simulink model "mpsk"  (Simulink 6.4)
settings: Solver=FixedStepDiscrete  StartTime=0.0  StopTime=inf  RelTol=1e-3
libraries: commsink2 x2, commdigbbndpm3 x2, commchan3 x1, commrandsrc2 x1
settings Model: Creator=ALEX  LastModifiedBy=student
settings OptimizationCC: InitFltsAndDblsToZero=off
settings DebuggingCC: SignalResolutionControl=UseLocalSettings  MultiTaskDSMMsg=error  MultiTaskCondExecSysMsg=error
settings GRTTargetCC: TargetFcnLib=ansi_tfl_table_tmw.mat

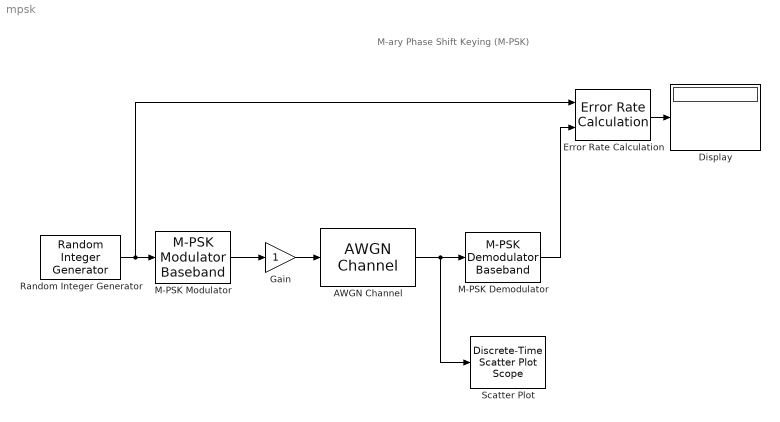
== system mpsk ==
  note: M-ary Phase Shift Keying (M-PSK)
  AWGN Channel : commchan3/AWGN Channel  SystemSampleTime=-1  seed=67  noiseMode="Signal to noise ratio  (Es/No)"  EbNodB=3  EsNodB=100  SNRdB=10  bitsPerSym=1  Ps=1  Tsym=1  variance=0.1
  Display : Display
  Error Rate Calculation : commsink2/Error Rate Calculation  N=0  st_delay=0  cp_mode=Entire frame  subframe=[]  PMode=Port  WsName=ErrorVec  RsMode2=off  stop=off  numErr=10000  maxBits=100000
  Gain : Gain  ParameterDataType=fixdt(1, 16)  OutDataType=fixdt(1, 16)
  M-PSK Demodulator : commdigbbndpm3/M-PSK Demodulator Baseband  M=8  OutType=Integer  Dec=Binary  Mapping=[0:7]  Ph=0  outDtype1=int8  outDtype2=int8
  M-PSK Modulator : commdigbbndpm3/M-PSK Modulator Baseband  M=8  InType=Integer  Enc=Binary  Mapping=[0:7]  Ph=0  outDtype=double  outWordLen=16  outUDDataType=sfix(16)  outFracLenMode=Best precision  outFracLen=15
  Random Integer Generator : commrandsrc2/Random Integer Generator  SystemSampleTime=-1  mul=8  seed=37  Ts=1  frameBased=off  sampPerFrame=8  orient=off  outDataType=int8
  Scatter Plot : commsink2/Discrete-Time Scatter Plot Scope  Tag=ScatterPlot  SystemSampleTime=-1  sampPerSymb=1  offsetEye=0  numTraces=100  numNewFrames=10  LineMarkers=.  LineColors=b  fading=on  render=on  AxisGrid=on  xMin=-2  xMax=2  yMin=-2  yMax=2  inphaseLabel=In-phase Amplitude  quadratureLabel=Quadrature Amplitude  openScopeAtSimStart=off  FrameNumber=off  FigPos=[360 435 560 487]  figTitle=Scatter Plot  numLinesMax=8  block_type_=scatter
  wires:
  Error Rate Calculation/1 -> Display/1
  Random Integer Generator/1 -> M-PSK Modulator/1, Error Rate Calculation/1
  M-PSK Modulator/1 -> Gain/1
  Gain/1 -> AWGN Channel/1
  AWGN Channel/1 -> M-PSK Demodulator/1, Scatter Plot/1
  M-PSK Demodulator/1 -> Error Rate Calculation/2
